simulink model "sampleModel1614_sub_sub"  (R2023a)
settings: Solver=VariableStepAuto  StartTime=0.0  StopTime=10.0  RelTol=1e-3
libraries: hdlsllib x3
settings Model: Creator=user1  LastModifiedBy=user1
settings OptimizationCC: BlockReduction=off  ConditionallyExecuteInputs=off

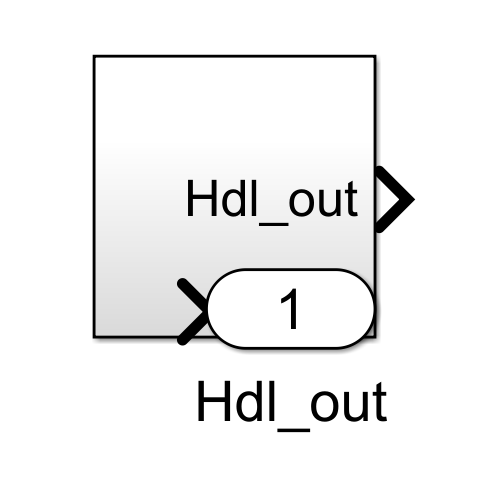
[thumbnail: Simulink's stored preview of the top-level diagram]
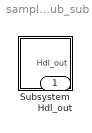
== system sampleModel1614_sub_sub ==
  Subsystem : Subsystem
  Hdl_out : Outport  OutDataTypeStr=uint8

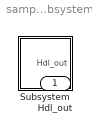
== system sampleModel1614_sub_sub/Subsystem ==
  Subsystem : Subsystem
  Hdl_out : Outport  OutDataTypeStr=uint8

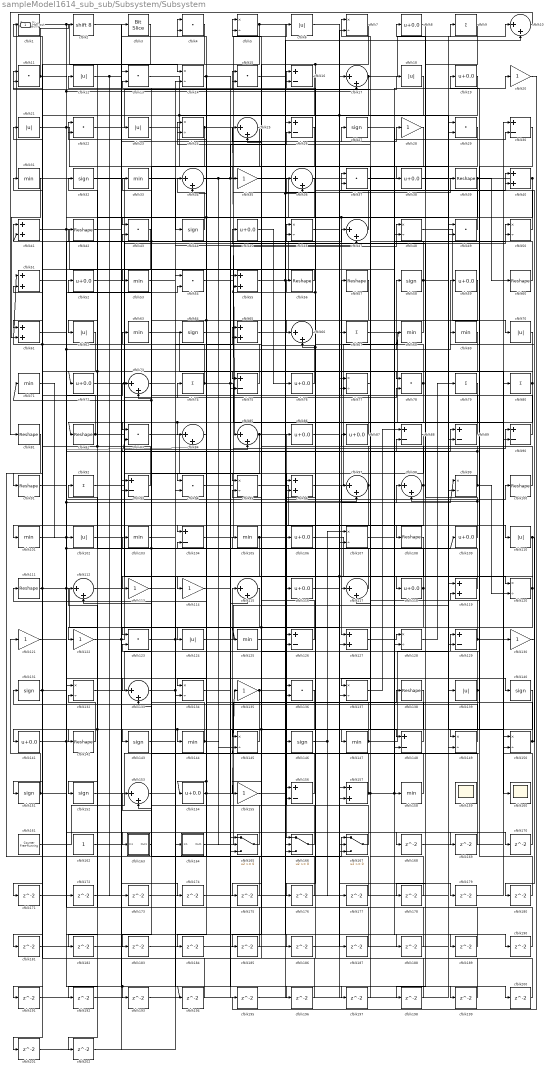
== system sampleModel1614_sub_sub/Subsystem/Subsystem ==
  cfblk1 : hdlsllib/Logic and Bit Operations/Detect Rise Nonnegative  vinit=0  OutDataTypeStr=uint8
  cfblk{10,17,25,34,36,47,66,73,84..85,97..98,112,115,117,133,153} (17 alike) : Sum  Inputs=|++  OutDataTypeStr=uint8
  cfblk{39,42,56..57,60,81..82,91,100,108,111,138,142} (13 alike) : Reshape
  cfblk{31,33,53,63,68..69,71,101,103,105,125,144,147,158} (14 alike) : MinMax  OutDataTypeStr=uint8
  cfblk{6,12,18,21,23,62,70,102,110,124,139} (11 alike) : Abs  OutDataTypeStr=uint8  SaturateOnIntegerOverflow=off
  cfblk{16,26,30,75,88..90,93,104,126,129,148,156} (13 alike) : Sum  Inputs=+-  OutDataTypeStr=uint8
  cfblk{8,19,38,45,52,59,72,76,86..87,106,109,116,118,141,154} (16 alike) : Bias  Bias=0.0  SaturateOnIntegerOverflow=off
  cfblk{5,7,14,24,46,48,50,77,95,99,107,120,128,132,134,137,145,149..150} (19 alike) : Product  Inputs=*/  OutDataTypeStr=uint8  RndMeth=Zero  SaturateOnIntegerOverflow=on
  cfblk{4,11,13,15,22,29,37,43,49,54,78,83,94,123,136} (15 alike) : DotProduct  OutDataTypeStr=uint8
  cfblk{20,28,35,113..114,121..122,130,135,155} (10 alike) : Gain  OutDataTypeStr=uint8
  cfblk{40..41,51,55,61,65,96,119,127,157} (10 alike) : Sum  OutDataTypeStr=uint8
  cfblk{27,32,44,58,64,131,140,143,146,151..152} (11 alike) : Signum
  cfblk159 : Scope
      settings: Floating=on
  cfblk160 : Scope
  cfblk161 : hdlsllib/Sources/Counter Free-Running  NumBits=16  tsamp=-1
  cfblk162 : Constant  OutDataTypeStr=uint8  SampleTime=-1
  cfblk163 : Subsystem
      settings: LibrarySourceBlock=|
      | hdlsllib/Ports &
      | Subsystems/Subsystem
  cfblk164 : Subsystem
      settings: LibrarySourceBlock=|
      | hdlsllib/Ports &
      | Subsystems/Subsystem
  cfblk165 : Switch  OutDataTypeStr=uint8  SaturateOnIntegerOverflow=off  InputSameDT=off
  cfblk166 : Switch  OutDataTypeStr=uint8  SaturateOnIntegerOverflow=off  InputSameDT=off
  cfblk167 : Switch  OutDataTypeStr=uint8  SaturateOnIntegerOverflow=off  InputSameDT=off
  cfblk{168..202} (35 alike) : Delay  SampleTime=1
  cfblk2 : ArithShift  BitShiftNumber=8
  cfblk3 : hdlsllib/Logic and Bit Operations/Bit Slice  lidx=7  ridx=0
  cfblk{9,67,74,79..80,92} (6 alike) : Sum  Inputs=+  OutDataTypeStr=uint8
  Hdl_out : Outport  OutDataTypeStr=uint8
  wires:
  cfblk202/1 -> cfblk23/1
  cfblk201/1 -> cfblk14/2
  cfblk200/1 -> cfblk96/2
  cfblk199/1 -> cfblk1/1
  cfblk198/1 -> cfblk95/2
  cfblk69/1 -> cfblk198/1
  cfblk197/1 -> cfblk37/2
  cfblk51/1 -> cfblk197/1
  cfblk196/1 -> cfblk54/1
  cfblk64/1 -> cfblk196/1
  cfblk195/1 -> cfblk156/1
  cfblk20/1 -> cfblk195/1
  cfblk194/1 -> cfblk11/2
  cfblk193/1 -> cfblk115/2
  cfblk192/1 -> cfblk149/2
  cfblk191/1 -> cfblk157/1
  cfblk190/1 -> cfblk165/1
  cfblk189/1 -> cfblk13/1
  cfblk65/1 -> cfblk189/1
  cfblk188/1 -> cfblk117/2
  cfblk187/1 -> cfblk112/1
  cfblk186/1 -> cfblk17/1
  cfblk143/1 -> cfblk186/1
  cfblk185/1 -> cfblk132/1
  cfblk184/1 -> cfblk77/2
  cfblk183/1 -> cfblk49/2
  cfblk182/1 -> cfblk7/2
  cfblk181/1 -> cfblk126/1
  cfblk180/1 -> cfblk119/2
  cfblk179/1 -> cfblk150/1
  cfblk6/1 -> cfblk179/1
  cfblk178/1 -> cfblk97/1
  cfblk8/1 -> cfblk178/1
  cfblk177/1 -> cfblk5/2
  cfblk176/1 -> cfblk34/2
  cfblk175/1 -> cfblk153/1
  cfblk18/1 -> cfblk175/1
  cfblk174/1 -> cfblk16/2
  cfblk2/1 -> cfblk174/1
  cfblk173/1 -> cfblk29/2
  cfblk172/1 -> cfblk89/2
  cfblk61/1 -> cfblk172/1
  cfblk171/1 -> cfblk94/2
  cfblk43/1 -> cfblk171/1
  cfblk170/1 -> cfblk30/1
  cfblk116/1 -> cfblk170/1
  cfblk169/1 -> cfblk123/2
  cfblk152/1 -> cfblk169/1
  cfblk168/1 -> cfblk90/2
  cfblk86/1 -> cfblk168/1
  cfblk119/1 -> cfblk15/1
  cfblk110/1 -> cfblk166/3, cfblk157/2, cfblk180/1
  cfblk166/1 -> cfblk22/2
  cfblk12/1 -> cfblk93/1, cfblk173/1
  cfblk129/1 -> cfblk80/1, cfblk15/2
  cfblk66/1 -> cfblk96/1
  cfblk42/1 -> cfblk27/1
  cfblk59/1 -> cfblk166/2
  cfblk100/1 -> cfblk43/2
  cfblk130/1 -> cfblk40/2
  cfblk15/1 -> cfblk97/2
  cfblk19/1 -> cfblk75/1, cfblk167/3
  cfblk75/1 -> cfblk4/2
  cfblk70/1 -> cfblk152/1
  cfblk30/1 -> cfblk149/1
  cfblk113/1 -> cfblk28/1
  cfblk34/1 -> cfblk167/2, cfblk26/2, cfblk145/2
  cfblk79/1 -> cfblk116/1
  cfblk146/1 -> cfblk107/1, cfblk177/1
  cfblk148/1 -> cfblk66/2, cfblk36/1
  cfblk35/1 -> cfblk119/1
  cfblk16/1 -> cfblk141/1
  cfblk50/1 -> cfblk8/1
  cfblk26/1 -> cfblk156/2
  cfblk106/1 -> cfblk120/1
  cfblk93/1 -> cfblk32/1, cfblk31/1
  cfblk155/1 -> cfblk138/1
  cfblk38/1 -> cfblk150/2
  cfblk157/1 -> cfblk87/1, cfblk20/1, cfblk106/1
  cfblk135/1 -> cfblk10/2, cfblk183/1
  cfblk165/1 -> cfblk112/2
  cfblk13/1 -> cfblk77/1, cfblk99/2
  cfblk78/1 -> cfblk55/2, cfblk41/1, cfblk93/2
  cfblk114/1 -> cfblk48/1
  cfblk121/1 -> cfblk88/2, cfblk99/1
  cfblk162/1 -> cfblk4/1
  cfblk120/1 -> cfblk125/1, cfblk155/1, cfblk113/1
  cfblk37/1 -> cfblk30/2
  cfblk108/1 -> cfblk153/2
  cfblk105/1 -> cfblk26/1, cfblk134/2
  cfblk153/1 -> cfblk89/1
  cfblk5/1 -> cfblk137/2, cfblk36/2, cfblk91/1
  cfblk56/1 -> cfblk53/1
  cfblk52/1 -> cfblk85/2
  cfblk76/1 -> cfblk25/1
  cfblk46/1 -> cfblk110/1
  cfblk33/1 -> cfblk44/1
  cfblk4/1 -> cfblk122/1, cfblk72/1
  cfblk85/1 -> cfblk143/1, cfblk107/2
  cfblk133/1 -> cfblk65/2, cfblk200/1
  cfblk58/1 -> cfblk137/1, cfblk24/2, cfblk10/1
  cfblk123/1 -> cfblk164/1(In1), cfblk98/1
  cfblk131/1 -> cfblk54/2, cfblk201/1
  cfblk163/1(Out1) -> cfblk13/2
  cfblk7/1 -> cfblk145/1, cfblk176/1
  cfblk29/1 -> cfblk117/1
  cfblk112/1 -> cfblk40/1
  cfblk126/1 -> cfblk5/1
  cfblk118/1 -> cfblk127/2, cfblk25/2
  cfblk124/1 -> cfblk49/1
  cfblk80/1 -> cfblk82/1, cfblk84/1, cfblk78/1
  cfblk67/1 -> cfblk129/2
  cfblk41/1 -> cfblk193/1, cfblk194/1, cfblk128/2
  cfblk73/1 -> cfblk47/2
  cfblk107/1 -> cfblk50/2
  cfblk62/1 -> cfblk151/1
  cfblk96/1 -> cfblk58/1
  cfblk49/1 -> cfblk37/1
  cfblk132/1 -> cfblk126/2
  cfblk81/1 -> cfblk167/1
  cfblk141/1 -> cfblk68/1, cfblk46/2, cfblk163/1(In1)
  cfblk164/1(Out1) -> cfblk67/1
  cfblk95/1 -> cfblk108/1
  cfblk11/1 -> cfblk17/2, cfblk133/1, cfblk2/1
  cfblk25/1 -> cfblk43/1
  cfblk89/1 -> cfblk57/1
  cfblk23/1 -> cfblk139/1
  cfblk99/1 -> cfblk56/1, cfblk83/2, cfblk120/2
  cfblk136/1 -> cfblk181/1, cfblk182/1
  cfblk147/1 -> cfblk29/1, cfblk24/1
  cfblk103/1 -> cfblk64/1
  cfblk9/1 -> cfblk38/1
  cfblk127/1 -> cfblk128/1
  cfblk97/1 -> cfblk16/1, cfblk165/3
  cfblk1/1 -> cfblk14/1, cfblk84/2
  cfblk83/1 -> cfblk136/2
  cfblk140/1 -> cfblk146/1
  cfblk125/1 -> cfblk136/1
  cfblk28/1 -> cfblk154/1, cfblk184/1
  cfblk91/1 -> cfblk140/1
  cfblk57/1 -> cfblk124/1, cfblk83/1
  cfblk134/1 -> cfblk55/1
  cfblk60/1 -> cfblk11/1
  cfblk154/1 -> cfblk135/1, cfblk104/2
  cfblk144/1 -> cfblk52/1, cfblk71/1, cfblk165/2
  cfblk87/1 -> cfblk22/1, cfblk41/2
  cfblk31/1 -> cfblk61/2
  cfblk3/1 -> cfblk61/1
  cfblk115/1 -> cfblk123/1
  cfblk98/1 -> cfblk101/1, cfblk42/1
  cfblk55/1 -> cfblk47/1, cfblk148/2
  cfblk158/1 -> cfblk65/1
  cfblk88/1 -> cfblk166/1
  cfblk92/1 -> cfblk95/1
  cfblk102/1 -> cfblk3/1
  cfblk150/1 -> cfblk59/1, cfblk7/1
  cfblk68/1 -> cfblk66/1
  cfblk48/1 -> cfblk70/1
  cfblk63/1 -> cfblk160/1
  cfblk22/1 -> cfblk18/1
  cfblk77/1 -> cfblk147/1
  cfblk109/1 -> cfblk45/1, cfblk98/2
  cfblk36/1 -> cfblk104/1, cfblk62/1
  cfblk139/1 -> cfblk105/1, cfblk19/1, cfblk202/1
  cfblk10/1 -> cfblk81/1
  cfblk167/1 -> cfblk86/1
  cfblk74/1 -> cfblk69/1, cfblk130/1, cfblk51/1, cfblk51/2
  cfblk90/1 -> cfblk33/1
  cfblk39/1 -> cfblk127/1, cfblk73/2, cfblk60/1
  cfblk72/1 -> cfblk50/1, cfblk78/2
  cfblk84/1 -> cfblk134/1
  cfblk21/1 -> cfblk35/1, cfblk48/2
  cfblk32/1 -> cfblk118/1
  cfblk117/1 -> cfblk92/1, cfblk63/1
  cfblk145/1 -> cfblk142/1
  cfblk27/1 -> cfblk158/1, cfblk190/1
  cfblk17/1 -> cfblk9/1, cfblk75/2
  cfblk47/1 -> cfblk12/1
  cfblk24/1 -> cfblk85/1, cfblk133/2
  cfblk142/1 -> cfblk132/2
  cfblk53/1 -> cfblk46/1
  cfblk94/1 -> cfblk90/1
  cfblk54/1 -> cfblk39/1
  cfblk111/1 -> cfblk73/1, cfblk109/1, cfblk187/1, cfblk191/1
  cfblk122/1 -> cfblk74/1, cfblk199/1
  cfblk101/1 -> cfblk100/1, cfblk188/1
  cfblk40/1 -> cfblk111/1, Hdl_out/1
  cfblk104/1 -> cfblk6/1
  cfblk44/1 -> cfblk34/1
  cfblk82/1 -> cfblk114/1, cfblk21/1
  cfblk14/1 -> cfblk94/1, cfblk148/1
  cfblk45/1 -> cfblk76/1
  cfblk151/1 -> cfblk121/1, cfblk103/1
  cfblk156/1 -> cfblk115/1
  cfblk128/1 -> cfblk79/1
  cfblk138/1 -> cfblk144/1, cfblk192/1, cfblk185/1
  cfblk71/1 -> cfblk102/1
  cfblk161/1 -> cfblk129/1
  cfblk149/1 -> cfblk131/1
  cfblk137/1 -> cfblk88/1

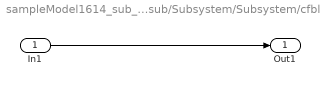
== system sampleModel1614_sub_sub/Subsystem/Subsystem/cfblk163 ==
  In1 : Inport
  Out1 : Outport
  wires:
  In1/1 -> Out1/1

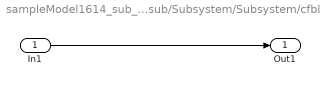
== system sampleModel1614_sub_sub/Subsystem/Subsystem/cfblk164 ==
  In1 : Inport
  Out1 : Outport
  wires:
  In1/1 -> Out1/1
